simulink model "Excess of Passivity Q3"  (R2021b)
settings: Solver=ode4  StartTime=0.0  StopTime=20  FixedStep=0.0001  RelTol=1e-3
libraries: slpidlib x2
settings Model: Creator=rmkna  LastModifiedBy=rmkna

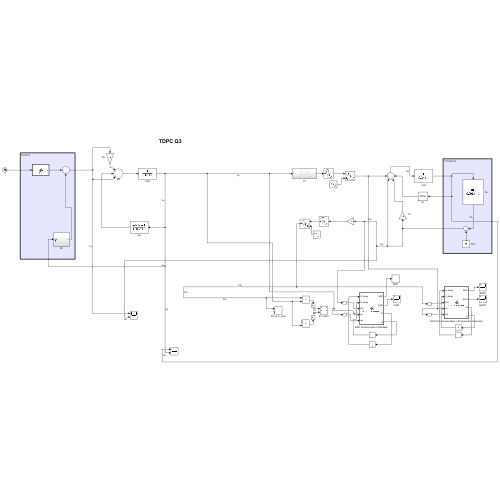
[thumbnail: Simulink's stored preview of the top-level diagram]
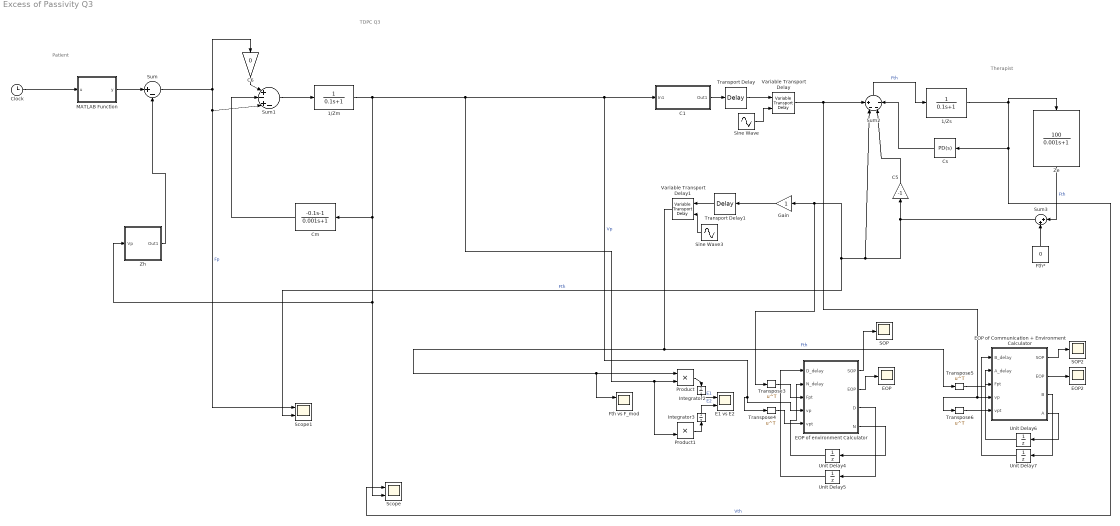
== system Excess of Passivity Q3 ==
  note: TDPC Q3
  note: Therapist
  note: Patient
  1/Zm : TransferFcn  Denominator=[0.1 1]
  1/Zs : TransferFcn  Denominator=[0.1 1]
  C1 : Subsystem
  "C5 " : Gain  Gain=-1
  "C6 " : Gain  Gain=0
  Clock : Clock
  Cm : TransferFcn  Numerator=[-0.1 -1]  Denominator=[0.001 1]
  Cs : slpidlib/PID Controller  Controller=PD  Form=Parallel  TimeDomain=Continuous-time  UseExternalTs=off  SampleTime=-1  IntegratorMethod=Forward Euler  FilterMethod=Forward Euler  ControllerParametersSource=internal  P=1000  I=1  D=1  UseFilter=on  N=1000  TunerSelectOption=Transfer Function Based (PID Tuner App)  InitialConditionSource=internal  InitialConditionForIntegrator=0  InitialConditionForFilter=0  DifferentiatorICPrevScaledInput=0  ExternalReset=none  TrackingMode=off  Kt=1  LimitOutput=off  SatLimitsSource=internal  UpperSaturationLimit=inf  LowerSaturationLimit=-inf  LinearizeAsGain=on  AntiWindupMode=none  Kb=1  POutMin=[]  POutMax=[]  IOutMin=[]  IOutMax=[]  DOutMin=[]  DOutMax=[]  NOutMin=[]  NOutMax=[]  SumOutMin=[]  SumOutMax=[]  SaturationOutMin=[]  SaturationOutMax=[]  PParamMin=[]  PParamMax=[]  IParamMin=[]  IParamMax=[]  DParamMin=[]  DParamMax=[]  NParamMin=[]  NParamMax=[]  KbParamMin=[]  KbParamMax=[]  KtParamMin=[]  KtParamMax=[]  KbOutMin=[]  KbOutMax=[]  KtOutMin=[]  KtOutMax=[]  IntegratorOutMin=[]  IntegratorOutMax=[]  FilterOutMin=[]  FilterOutMax=[]  SumI1OutMin=[]  SumI1OutMax=[]  SumI2OutMin=[]  SumI2OutMax=[]  SumI3OutMin=[]  SumI3OutMax=[]  SumI4OutMin=[]  SumI4OutMax=[]  SumDOutMin=[]  SumDOutMax=[]  DifferentiatorOutMin=[]  DifferentiatorOutMax=[]  FilterDiffOutCoefMin=[]  FilterDiffOutCoefMax=[]  ReciprocalOutMin=[]  ReciprocalOutMax=[]  SumDenOutMin=[]  SumDenOutMax=[]  SumNumOutMin=[]  SumNumOutMax=[]  DivideOutMin=[]  DivideOutMax=[]  UdiffTsProdOutMin=[]  UdiffTsProdOutMax=[]  NTsProdOutMin=[]  NTsProdOutMax=[]  UintegralTsProdOutMin=[]  UintegralTsProdOutMax=[]  UngainTsProdOutMin=[]  UngainTsProdOutMax=[]  IntegratorContinuousStateAttributes=''  IntegratorStateMustResolveToSignalObject=off  IntegratorRTWStateStorageClass=Auto  FilterContinuousStateAttributes=''  FilterStateMustResolveToSignalObject=off  FilterRTWStateStorageClass=Auto  ParallelPVariant=InternalParameters  IdealPVariant=Disabled  IVariant=Disabled  DVariant=InternalParameters  IntegratorVariant=Disabled  SatVariant=Disabled  AWVariant=Disabled  PCopyVariant=Disabled  TRVariant=Disabled  FdbkBlocksVariant=Forward  IdealPFdbkVariant=Disabled  SatFdbkVariant=Disabled  DerivativeFilterVariant=ContFilter  NVariant=InternalParameters  NCopyVariant=Disabled  FilterICVariant=InternalICsFilter  IntegratorICVariant=Disabled  ExternalResetVariant=Disabled  TRSumVariant=Passthrough  SumFdbkVariant=Disabled  SumVariant=Sum_PD  TsampFilterVariant=InternalTs  TsampNgainVariant=Passthrough  TsampIntegralVariant=Disabled_SignalSpec  ExternalSaturationOutDataTypeStr=Inherit: Same as second input
  E1 vs E2 : Scope  NumInputPorts=2
  EOP : Scope
  EOP of Communication + Environment Calculator : MATLAB Function  TreatAsAtomicUnit=on
  EOP of environment Calculator : MATLAB Function  TreatAsAtomicUnit=on
  EOP2 : Scope
  Fth vs F_mod : Scope  NumInputPorts=2
  Fth* : Constant  Value=0  OutDataTypeStr=Inherit: Inherit via back propagation
  Gain : Gain
  Integrator2 : Integrator
  Integrator3 : Integrator
  MATLAB Function : MATLAB Function  TreatAsAtomicUnit=on
  Product : Product
  Product1 : Product
  SOP : Scope
  SOP2 : Scope
  Scope : Scope  NumInputPorts=2
  Scope1 : Scope  NumInputPorts=2
  Sine Wave : Sin  Amplitude=0.02  Frequency=12  Phase=pi/2  SampleTime=0
  Sine Wave3 : Sin  Amplitude=0.02  Frequency=12  Phase=pi/2  SampleTime=0
  Sum : Sum  Inputs=|+-
  Sum1 : Sum  Inputs=|+-+-
  Sum2 : Sum  Inputs=+---
  Sum3 : Sum  Inputs=|++
  Transport Delay : TransportDelay  DelayTime=0.1  PadeOrder=3
  Transport Delay1 : TransportDelay  DelayTime=0.1  PadeOrder=3
  Transpose{3..6} (4 alike) : Math  Operator=transpose  SaturateOnIntegerOverflow=on
  Unit Delay{4..7} (4 alike) : UnitDelay  SampleTime=-1  HasFrameUpgradeWarning=on
  Variable Transport Delay : VariableTransportDelay  PadeOrder=3
  Variable Transport Delay1 : VariableTransportDelay  PadeOrder=3
  Ze : TransferFcn  Numerator=[100]  Denominator=[0.001 1]
  Zh : Subsystem
  wires:
  MATLAB Function/1(y) -> Sum/1
  Sine Wave3/1 -> Variable Transport Delay1/2
  EOP of Communication + Environment Calculator/1(SOP) -> SOP2/1
  EOP of Communication + Environment Calculator/2(EOP) -> EOP2/1
  Transpose4/1 -> EOP of environment Calculator/5(vpt)
  Transpose5/1 -> EOP of Communication + Environment Calculator/3(Fpt)
  EOP of Communication + Environment Calculator/4(A) -> Unit Delay6/1
  Sum1/1 -> 1/Zm/1
  Transport Delay1/1 -> Variable Transport Delay1/1
  EOP of environment Calculator/3(D) -> Unit Delay5/1
  Unit Delay6/1 -> EOP of Communication + Environment Calculator/2(A_delay)
  EOP of Communication + Environment Calculator/3(B) -> Unit Delay7/1
  Transpose6/1 -> EOP of Communication + Environment Calculator/5(vpt)
  EOP of environment Calculator/4(N) -> Unit Delay4/1
  1/Zm/1 -> Scope/2, Zh/1(Vp), Cm/1, Product1/2, Product/2, EOP of environment Calculator/4(vp), Transpose4/1, C1/1(In1)  "Vp"
  Unit Delay4/1 -> EOP of environment Calculator/2(N_delay)
  Unit Delay7/1 -> EOP of Communication + Environment Calculator/1(B_delay)
  Sine Wave/1 -> Variable Transport Delay/2
  Integrator2/1 -> E1 vs E2/1  "E1"
  Sum3/1 -> Scope1/2, Gain/1, Transpose3/1, Sum2/2, "C5 "/1  "Fth"
  Integrator3/1 -> E1 vs E2/2  "E2"
  Product1/1 -> Integrator3/1
  Product/1 -> Integrator2/1
  EOP of environment Calculator/1(SOP) -> SOP/1
  1/Zs/1 -> Scope/1, Cs/1, Ze/1  "Vth"
  Variable Transport Delay/1 -> Transpose6/1, EOP of Communication + Environment Calculator/4(vp), Sum2/1
  Transpose3/1 -> EOP of environment Calculator/3(Fpt)
  Unit Delay5/1 -> EOP of environment Calculator/1(D_delay)
  C1/1(Out1) -> Transport Delay/1
  EOP of environment Calculator/2(EOP) -> EOP/1
  Variable Transport Delay1/1 -> Transpose5/1, Fth vs F_mod/1, Product/1  "Fth"
  Sum/1 -> Scope1/1, Sum1/3, "C6 "/1  "Fp"
  "C5 "/1 -> Sum2/3
  Cm/1 -> Sum1/2
  Transport Delay/1 -> Variable Transport Delay/1
  Sum2/1 -> 1/Zs/1  "Fth"
  Fth*/1 -> Sum3/2
  "C6 "/1 -> Sum1/1
  Ze/1 -> Sum3/1  "Fth"
  Clock/1 -> MATLAB Function/1(u)
  Zh/1(Out1) -> Sum/2
  Gain/1 -> Transport Delay1/1
  Cs/1 -> Sum2/4

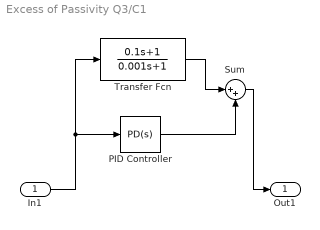
== system Excess of Passivity Q3/C1 ==
  In1 : Inport
  PID Controller : slpidlib/PID Controller  Controller=PD  Form=Parallel  TimeDomain=Continuous-time  UseExternalTs=off  SampleTime=-1  IntegratorMethod=Forward Euler  FilterMethod=Forward Euler  ControllerParametersSource=internal  P=1000  I=1  D=1  UseFilter=on  N=1000  TunerSelectOption=Transfer Function Based (PID Tuner App)  InitialConditionSource=internal  InitialConditionForIntegrator=0  InitialConditionForFilter=0  DifferentiatorICPrevScaledInput=0  ExternalReset=none  TrackingMode=off  Kt=1  LimitOutput=off  SatLimitsSource=internal  UpperSaturationLimit=inf  LowerSaturationLimit=-inf  LinearizeAsGain=on  AntiWindupMode=none  Kb=1  POutMin=[]  POutMax=[]  IOutMin=[]  IOutMax=[]  DOutMin=[]  DOutMax=[]  NOutMin=[]  NOutMax=[]  SumOutMin=[]  SumOutMax=[]  SaturationOutMin=[]  SaturationOutMax=[]  PParamMin=[]  PParamMax=[]  IParamMin=[]  IParamMax=[]  DParamMin=[]  DParamMax=[]  NParamMin=[]  NParamMax=[]  KbParamMin=[]  KbParamMax=[]  KtParamMin=[]  KtParamMax=[]  KbOutMin=[]  KbOutMax=[]  KtOutMin=[]  KtOutMax=[]  IntegratorOutMin=[]  IntegratorOutMax=[]  FilterOutMin=[]  FilterOutMax=[]  SumI1OutMin=[]  SumI1OutMax=[]  SumI2OutMin=[]  SumI2OutMax=[]  SumI3OutMin=[]  SumI3OutMax=[]  SumI4OutMin=[]  SumI4OutMax=[]  SumDOutMin=[]  SumDOutMax=[]  DifferentiatorOutMin=[]  DifferentiatorOutMax=[]  FilterDiffOutCoefMin=[]  FilterDiffOutCoefMax=[]  ReciprocalOutMin=[]  ReciprocalOutMax=[]  SumDenOutMin=[]  SumDenOutMax=[]  SumNumOutMin=[]  SumNumOutMax=[]  DivideOutMin=[]  DivideOutMax=[]  UdiffTsProdOutMin=[]  UdiffTsProdOutMax=[]  NTsProdOutMin=[]  NTsProdOutMax=[]  UintegralTsProdOutMin=[]  UintegralTsProdOutMax=[]  UngainTsProdOutMin=[]  UngainTsProdOutMax=[]  IntegratorContinuousStateAttributes=''  IntegratorStateMustResolveToSignalObject=off  IntegratorRTWStateStorageClass=Auto  FilterContinuousStateAttributes=''  FilterStateMustResolveToSignalObject=off  FilterRTWStateStorageClass=Auto  ParallelPVariant=InternalParameters  IdealPVariant=Disabled  IVariant=Disabled  DVariant=InternalParameters  IntegratorVariant=Disabled  SatVariant=Disabled  AWVariant=Disabled  PCopyVariant=Disabled  TRVariant=Disabled  FdbkBlocksVariant=Forward  IdealPFdbkVariant=Disabled  SatFdbkVariant=Disabled  DerivativeFilterVariant=ContFilter  NVariant=InternalParameters  NCopyVariant=Disabled  FilterICVariant=InternalICsFilter  IntegratorICVariant=Disabled  ExternalResetVariant=Disabled  TRSumVariant=Passthrough  SumFdbkVariant=Disabled  SumVariant=Sum_PD  TsampFilterVariant=InternalTs  TsampNgainVariant=Passthrough  TsampIntegralVariant=Disabled_SignalSpec  ExternalSaturationOutDataTypeStr=Inherit: Same as second input
  Sum : Sum  Inputs=|++
  Transfer Fcn : TransferFcn  Numerator=[0.1 1]  Denominator=[0.001 1]
  Out1 : Outport
  wires:
  In1/1 -> PID Controller/1, Transfer Fcn/1
  Transfer Fcn/1 -> Sum/1
  PID Controller/1 -> Sum/2
  Sum/1 -> Out1/1

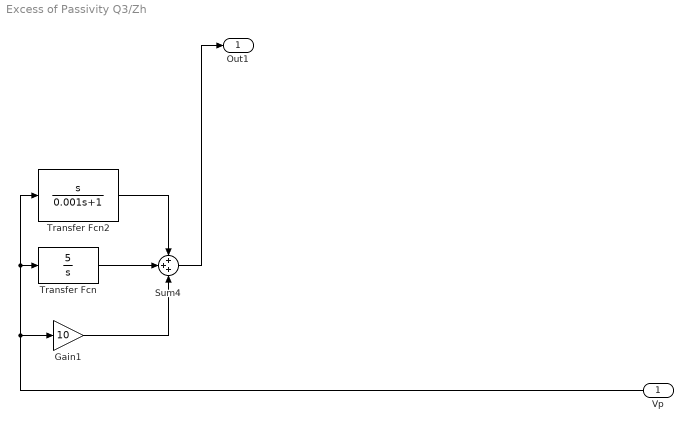
== system Excess of Passivity Q3/Zh ==
  Vp : Inport
  Gain1 : Gain  Gain=10
  Sum4 : Sum  Inputs=3
  Transfer Fcn : TransferFcn  Numerator=[5]  Denominator=[1 0]
  Transfer Fcn2 : TransferFcn  Numerator=[1 0]  Denominator=[0.001 1]
  Out1 : Outport
  wires:
  Vp/1 -> Gain1/1, Transfer Fcn/1, Transfer Fcn2/1
  Sum4/1 -> Out1/1
  Transfer Fcn/1 -> Sum4/2
  Transfer Fcn2/1 -> Sum4/1
  Gain1/1 -> Sum4/3

== matlab function Excess of Passivity Q3/EOP of environment Calculator ==
  data: D_delay input; N_delay input; SOP output; EOP output; Fpt input; vp input; vpt input; D output; N output
function [SOP,EOP,D,N] = EOP_Calculator(D_delay,N_delay,Fpt,vp,vpt)

N=N_delay+0.001*(Fpt*vp);
D=D_delay+0.001*(vpt*vp);
 
SOP= N/D;
 
EOP=-SOP;

== matlab function Excess of Passivity Q3/EOP of Communication + Environment Calculator ==
  data: B_delay input; A_delay input; SOP output; EOP output; Fpt input; vp input; vpt input; B output; A output
function [SOP,EOP,B,A] = EOP_Calculator(B_delay,A_delay,Fpt,vp,vpt)

A=A_delay+0.001*(Fpt*vp);
B=B_delay+0.001*(vpt*vp);
 
SOP=A/B;
 
EOP=-SOP;

== matlab function Excess of Passivity Q3/MATLAB Function ==
  data: u input; y output
function y = fcn(u)

y = sin(5*u)+ cos(8*u);
